simulink model "Mod5Counter"  (R2019b)
settings: Solver=VariableStepAuto  StartTime=0.0  StopTime=10.0  RelTol=1e-3
settings Model: Creator=ip  LastModifiedBy=ip

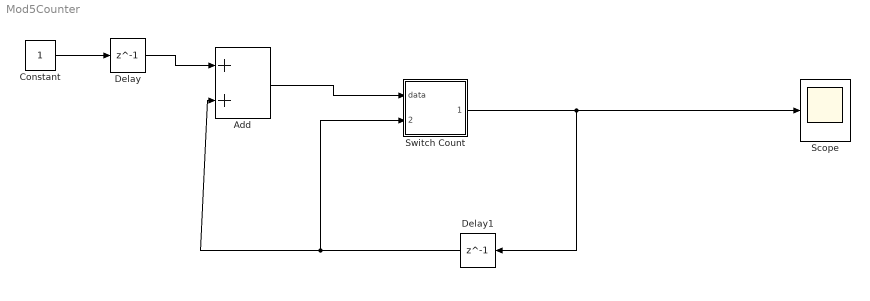
== system Mod5Counter ==
  Add : Sum
  Constant : Constant
  Delay : Delay  DelayLength=1
  Delay1 : Delay  DelayLength=1
  Scope : Scope
  Switch Count : Stateflow chart  BlockKeywords=__PRM__SERIALIZED__DATA__:Stateflow Chart,Stateflow Diagram  TreatAsAtomicUnit=on
  wires:
  Add/1 -> Switch Count/1(data)
  Constant/1 -> Delay/1
  Delay/1 -> Add/1
  Delay1/1 -> Switch Count/2(data1), Add/2
  Switch Count/1(data2) -> Delay1/1, Scope/1

== stateflow chart Mod5Counter/Switch Count ==
  (default) -> (junction 31)
  (junction 31) -> (junction 33) [order 1] : [feedback>=5]
  (junction 31) -> (junction 34) [order 2] : {output=input;}
  (junction 33) -> (junction 32) : {output=0;}
  (junction 32) -> (junction 34)
  (junction 34) -> (junction 35)
  data: data input; data1 input; data2 output
